simulink model "exp1"  (R2018a)
settings: Solver=VariableStepAuto  StartTime=0.0  StopTime=1.0  RelTol=1e-3
libraries: commchan3 x2, dsparch4 x2
settings Model: Creator=22121100  LastModifiedBy=22121100

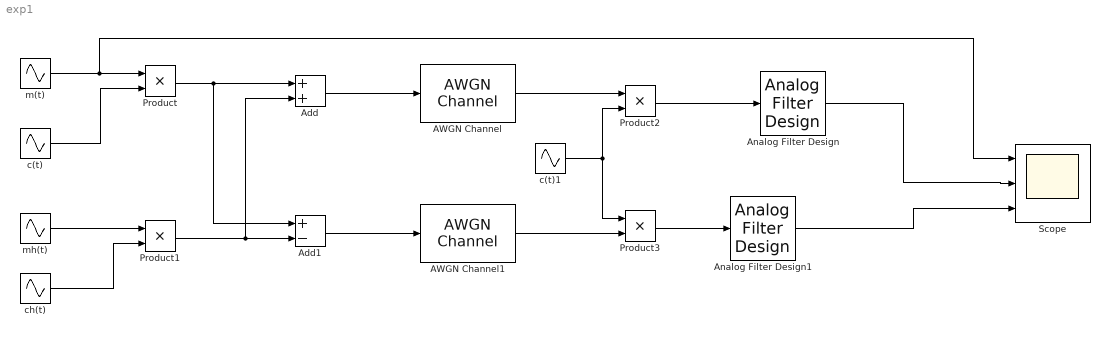
== system exp1 ==
  AWGN Channel : commchan3/AWGN Channel  InputProcessing=Columns as channels (frame based)  seed=67  noiseMode=Variance from mask  EbNodB=10  EsNodB=10  SNRdB=10  bitsPerSym=1  Ps=1  Tsym=1  variance=1
  AWGN Channel1 : commchan3/AWGN Channel  InputProcessing=Columns as channels (frame based)  seed=67  noiseMode=Variance from mask  EbNodB=10  EsNodB=10  SNRdB=10  bitsPerSym=1  Ps=1  Tsym=1  variance=1
  Add : Sum
  Add1 : Sum  Inputs=+-
  Analog Filter Design : dsparch4/Analog Filter Design  method=Butterworth  filttype=Lowpass  N=8  Wlo=5000  Whi=80  Rp=2  Rs=40
  Analog Filter Design1 : dsparch4/Analog Filter Design  method=Butterworth  filttype=Lowpass  N=8  Wlo=5000  Whi=80  Rp=2  Rs=40
  Product{,1..3} (4 alike) : Product
  Scope : Scope  NumInputPorts=3
  c(t) : Sin  Frequency=2*pi*5000  SampleTime=1/100000
  c(t)1 : Sin  Frequency=2*pi*5000  SampleTime=1/100000
  ch(t) : Sin  Frequency=2*pi*5000  SampleTime=1/100000
  m(t) : Sin  Frequency=2*pi*1000  Phase=pi/2  SampleTime=1/100000
  mh(t) : Sin  Frequency=2*pi*1000  SampleTime=1/100000
  wires:
  c(t)/1 -> Product/2
  mh(t)/1 -> Product1/1
  ch(t)/1 -> Product1/2
  Product1/1 -> Add/2, Add1/2
  Product/1 -> Add1/1, Add/1
  Add/1 -> AWGN Channel/1
  Add1/1 -> AWGN Channel1/1
  AWGN Channel/1 -> Product2/1
  Product2/1 -> Analog Filter Design/1
  c(t)1/1 -> Product3/1, Product2/2
  AWGN Channel1/1 -> Product3/2
  m(t)/1 -> Scope/1, Product/1
  Product3/1 -> Analog Filter Design1/1
  Analog Filter Design1/1 -> Scope/3
  Analog Filter Design/1 -> Scope/2
